simulink model "DRTelemedicine"  (R2026a)
settings: Solver=VariableStepDiscrete  StartTime=0  StopTime=params.simTimeMin * 60
values from neighbouring files (symbols this model uses):
  m = Simulink.Mask.get(blk)    [inspect_simevents_blocks.m]
  params = scenario_params('baseline')    [probe_bisect.m]    (also in probe_block_params.m = struct(          'meanArrivalTimeMin', 1.75,          'acqui; probe_diag.m; probe_full_vs_const.m; probe_inc.m = struct('meanArrivalTimeMin', 1.5,                  'acquisit)
settings Model: Creator=INSHRA SHAIKH  LastModifiedBy=INSHRA SHAIKH

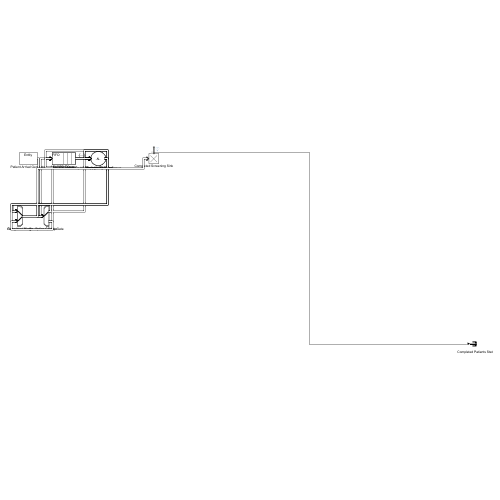
[thumbnail: Simulink's stored preview of the top-level diagram]
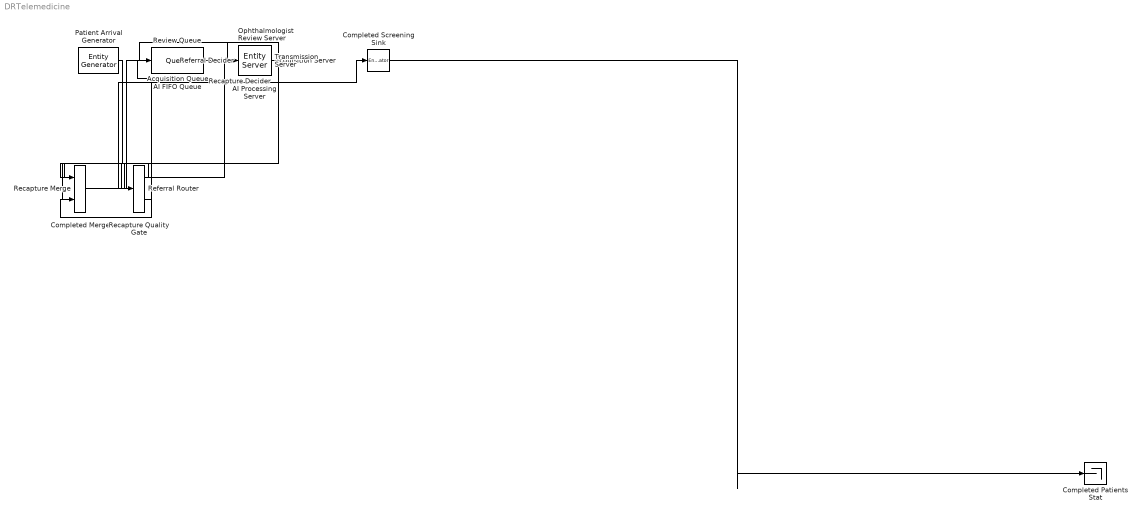
== system DRTelemedicine ==
  AI FIFO Queue : Queue  InputPortMessageModes=m  OutputPortMessageModes=m  Capacity=params.queueCapacity
  AI Processing Server : EntityServer  InputPortMessageModes=m  OutputPortMessageModes=m  Capacity=1  ServiceTimeValue=params.aiProcessTimeMin*60
  Acquisition Queue : Queue  InputPortMessageModes=m  OutputPortMessageModes=m  Capacity=params.acquisitionQueueCapacity
  Acquisition Server : EntityServer  InputPortMessageModes=m  OutputPortMessageModes=m  Capacity=1  ServiceTimeValue=params.acquisitionTimeMin*60
  Completed Merge : EntityInputSwitch  InputPortMessageModes=m,m  OutputPortMessageModes=m
  Completed Patients Stat : Terminator
  Completed Screening Sink : EntityTerminator  InputPortMessageModes=m  NumberEntitiesArrived=on
      settings: OutputPortMap=o0
  Ophthalmologist Review Server : EntityServer  InputPortMessageModes=m  OutputPortMessageModes=m  Capacity=params.numReviewers  ServiceTimeValue=params.reviewTimeMin*60
  Patient Arrival Generator : EntityGenerator  OutputPortMessageModes=m  TimeSource=MATLAB action  IntergenerationTimeAction=dt = -params.meanArrivalTimeMin*60*log(1-rand());  AttributeName=route  AttributeInitialValue=0  EntityType=Structured  EntityTypeName=Entity
  Recapture Decider : EntityServer  InputPortMessageModes=m  OutputPortMessageModes=m  Capacity=1  ServiceTimeValue=0  EntryAction=entity.route = 1 + double(rand() < params.recaptureRate);
  Recapture Merge : EntityInputSwitch  InputPortMessageModes=m,m  OutputPortMessageModes=m
  Recapture Quality Gate : EntityOutputSwitch  InputPortMessageModes=m  OutputPortMessageModes=m,m  SwitchingCriterion=From attribute  SwitchAttributeName=route
  Referral Decider : EntityServer  InputPortMessageModes=m  OutputPortMessageModes=m  Capacity=1  ServiceTimeValue=0  EntryAction=entity.route = 1 + double(rand() < params.referralRate);
  Referral Router : EntityOutputSwitch  InputPortMessageModes=m  OutputPortMessageModes=m,m  SwitchingCriterion=From attribute  SwitchAttributeName=route
  Review Queue : Queue  InputPortMessageModes=m  OutputPortMessageModes=m  Capacity=params.reviewQueueCapacity
  Transmission Server : EntityServer  InputPortMessageModes=m  OutputPortMessageModes=m  Capacity=1  ServiceTimeValue=params.transmissionDelayS + (params.imageSizeMB*8/params.bandwidthMbps)
  wires:
  Patient Arrival Generator/1 -> Recapture Merge/1
  Recapture Merge/1 -> Acquisition Queue/1
  Acquisition Queue/1 -> Acquisition Server/1
  Acquisition Server/1 -> Recapture Decider/1
  Recapture Decider/1 -> Recapture Quality Gate/1
  Recapture Quality Gate/1 -> Transmission Server/1
  Transmission Server/1 -> AI FIFO Queue/1
  AI FIFO Queue/1 -> AI Processing Server/1
  AI Processing Server/1 -> Referral Decider/1
  Referral Decider/1 -> Referral Router/1
  Referral Router/1 -> Completed Merge/1
  Referral Router/2 -> Review Queue/1
  Review Queue/1 -> Ophthalmologist Review Server/1
  Ophthalmologist Review Server/1 -> Completed Merge/2
  Completed Merge/1 -> Completed Screening Sink/1
  Recapture Quality Gate/2 -> Recapture Merge/2
  Completed Screening Sink/1 -> Completed Patients Stat/1
